simulink library "thermochemical"  (R2017b)
settings: Solver=VariableStepAuto  StartTime=0.0  StopTime=10.0  RelTol=1e-3
values from neighbouring files (symbols this model uses):
  c = conversion_factors()    [blk_clausius_clapeyron.m]    (also in blk_clausius_clapeyron_no_popup.m; blk_cold_room_closed_dry_air.m; blk_reactor_BaCl2_NH3_no_walls.m; blk_reactor_BaCl2_NH3_no_walls_state_space.m)
  cp = metal.cp    [blk_wall_simple.m]    (also in get_metal_properties.m = 390)
  fluid = get_param(blk,'fluid')    [blk_thermodynamic_properties_nonsaturated.m]    (also in blk_thermodynamic_properties_nonsaturated_interpreted.m; blk_thermodynamic_properties_saturated.m; blk_thermodynamic_properties_saturated_interpreted.m; blk_thermodynamic_properties_saturated_mix.m)
  gas = get_material_properties(x.gasName)    [blk_reactor_BaCl2_NH3_cylindrical_no_walls_fun1.m]
  h = get_param(gcb,'ObjectParameters')    [get_param_eval.m]
  rho = metal.rho    [blk_wall_simple.m]    (also in get_metal_properties.m = 8940)
  s = solve(eq,dx,'ReturnConditions',true)    [LMTD_inv.m]    (also in blk_wall_simple.m = get_param_eval(blk,'s'))
  u_gas_at_T_ref = -R * T_ref    [blk_reactor_BaCl2_NH3_no_walls.m]    (also in blk_reactor_BaCl2_NH3_no_walls_state_space.m)
undefined symbols (not defined in the file or in its folder): b_motor, BaCl2, beta, CoolProp, cP_binder, cP_gas, cP_s0, cv, dh_r_0, ENG, heat_exchanger_epsilonNTU_inv_simulink, heat_exchanger_epsilonNTU_simulink, J_motor, K_cin, kappa, Km_motor, La_motor, lookup2D_BreakPoint2, M_binder, N_binder, N_gas_free_volume_init, N_salt, NH3, nh3_v3, nu, P, phase, PID_D_motor, PID_I_motor, PID_P_motor, Ra_motor, Reactor_phase, T, T1, T2, T_init, Tr_init, Tr_ref, U_binder_at_Tr_ref, U_salt_at_X0_Tr_ref, Ur_init, V_void, Valve_regime, Vmax_motor, w_init_motor, X_init
libraries: thermochemical x247, simulink x54, dspsigops x3
(part 8 of 12)

== system thermochemical/Thermodynamic fluid properties/Thermodynamic property (non-saturated) (it uses CoolProp library)/Subsystem1 ==
  In1 : Inport
  In2 : Inport  Port=2
  Constant2 : Constant  Value=str2num(reciprocVar)
  CoolProp_function_call : MATLABFcn  MATLABFcn=CoolProp.PropsSI('Dmolar','T',u(1),'P',u(2)*100000,'Ammonia');
  Math Function : Math  Operator=reciprocal  SaturateOnIntegerOverflow=on
  Mux1 : Mux  Inputs=2
  switch2 : Switch  Criteria=u2 > Threshold
  Out1 : Outport
  wires:
  In2/1 -> Mux1/2
  In1/1 -> Mux1/1
  switch2/1 -> Out1/1
  Math Function/1 -> switch2/1
  Constant2/1 -> switch2/2
  CoolProp_function_call/1 -> Math Function/1, switch2/3
  Mux1/1 -> CoolProp_function_call/1

== system thermochemical/Thermodynamic fluid properties/Thermodynamic property (saturated)/Subsystem1 ==
  In1 : Inport
  look-up table 1D : Lookup_n-D  NumberOfTableDimensions=1  BreakpointsForDimension1=lookup1D_BreakPoint1  BreakpointsForDimension2=lookup2D_BreakPoint2  BreakpointsForDimension3=[5, 7]  BeginIndexSearchUsingPreviousIndexResult=on  Table=lookup1D_Data  ExtrapMethod=Clip  InternalRulePriority=Speed  RndMeth=Simplest  InputSameDT=on
  Out1 : Outport
  wires:
  In1/1 -> look-up table 1D/1
  look-up table 1D/1 -> Out1/1

== system thermochemical/Thermodynamic fluid properties/Thermodynamic property (saturated) (it uses CoolProp library)/Subsystem1 ==
  In1 : Inport
  Constant2 : Constant  Value=str2num(reciprocVar)
  CoolProp_function_call : MATLABFcn  MATLABFcn=CoolProp.PropsSI('P','T',u(1),'Q',0.5,'Ammonia')*1e-05;
  Math Function : Math  Operator=reciprocal  SaturateOnIntegerOverflow=on
  switch2 : Switch  Criteria=u2 > Threshold
  Out1 : Outport
  wires:
  In1/1 -> CoolProp_function_call/1
  switch2/1 -> Out1/1
  Math Function/1 -> switch2/1
  Constant2/1 -> switch2/2
  CoolProp_function_call/1 -> Math Function/1, switch2/3

== system thermochemical/Thermodynamic fluid properties/Thermodynamic property (saturated vapor-liquid mix)/Subsystem1 ==
  T(K) : Inport
  vapor quality (0..1) : Inport  Port=2
  1 : Constant
  Product : Product
  Product1 : Product
  Sum1 : Sum  Inputs=-+|
  Sum2 : Sum
  look-up table 1D : Lookup_n-D  NumberOfTableDimensions=1  BreakpointsForDimension1=fluid.sat.T  BreakpointsForDimension2=lookup2D_BreakPoint2  BreakpointsForDimension3=[5, 7]  BeginIndexSearchUsingPreviousIndexResult=on  Table=lookup1D_Data1  ExtrapMethod=Clip  InternalRulePriority=Speed  RndMeth=Simplest  InputSameDT=on
  look-up table 1D1 : Lookup_n-D  NumberOfTableDimensions=1  BreakpointsForDimension1=fluid.sat.T  BreakpointsForDimension2=lookup2D_BreakPoint2  BreakpointsForDimension3=[5, 7]  BeginIndexSearchUsingPreviousIndexResult=on  Table=lookup1D_Data2  ExtrapMethod=Clip  InternalRulePriority=Speed  RndMeth=Simplest  InputSameDT=on
  Out1 : Outport
  wires:
  Product1/1 -> Sum2/2
  1/1 -> Sum1/2
  Sum2/1 -> Out1/1
  Sum1/1 -> Product1/2  "1-Q"
  T(K)/1 -> look-up table 1D/1, look-up table 1D1/1
  look-up table 1D/1 -> Product1/1  "liquid"
  vapor quality (0..1)/1 -> Sum1/1, Product/2
  look-up table 1D1/1 -> Product/1  "vapor"
  Product/1 -> Sum2/1

== system thermochemical/Valves/Valve, gas, IEC 60534-2-1:2012 (exact)/Flow computation for compressible fluids, IEC 60534-2-1:2012 ==
  note: Valve flow model for compressible fluid,
      | according to IEC 60534-2-1:2012
  note: NOTE 2: for the 'regime' output to work properly, the model defines an enumerated type. This is done
      | inside the LoadFnc Callback of the model. (right click on the model -> Properties -> 'Callbacks' tab).
      | The enumerated type defined is the following:
      | Simulink.defineIntEnumType('Valve_regime',{'Open_NonChocked','Closed','Open_Chocked'},[1 0 -1])
  note: NOTE 1: Enumerations and Scopes
      | When a Scope block displays an enumerated signal, the vertical axis displays the names of
      | the enumerated values only if the scope was open during simulation. If you open the Scope
      | block for the first time before any simulation has occurred, or between simulations, the block
      | displays only numeric values.
  In1 : Inport
  In2 : Inport  Port=2
  In3 : Inport  Port=3
  In4 : Inport  Port=4
  In5 : Inport  Port=5
  Constant : Constant  Value=27.3
  Dead Zone : DeadZone  LowerValue=-Inf  UpperValue=1e-7  SaturateOnIntegerOverflow=on
  Display3 : Display
  Divide1 : Product  Inputs=***
  Divide2 : Product  Inputs=**
  Divide5 : Product  Inputs=***
  Sqrt : Sqrt  SaturateOnIntegerOverflow=on
  Subsystem : Subsystem
  Subsystem1 : Subsystem
  Valve regime : Subsystem
  Out1 : Outport
  Out2 : Outport  Port=2
  wires:
  Subsystem/1(non-chocked) -> Valve regime/2(In2)
  Divide2/1 -> Out1/1  "W (kg/h)"
  Sqrt/1 -> Divide2/2
  Divide1/1 -> Sqrt/1
  In5/1 -> Divide1/3  "rho upstream (kg/m3)"
  Divide5/1 -> Divide2/1  "N6 * Cv * Y"
  Constant/1 -> Divide5/3
  Subsystem1/1(Y) -> Divide5/2
  In1/1 -> Divide5/1, Dead Zone/1  "Cv"
  Subsystem/3(non-chocked1) -> Subsystem1/2(In2)
  Subsystem/2(non-chocked2) -> Divide1/1, Subsystem1/1(In1)  "x sizing"
  In2/1 -> Subsystem/3(P upstream (bar)1)  "gamma upstream (1)"
  In3/1 -> Subsystem/2(P upstream (bar)), Divide1/2  "P upstream (bar)"
  In4/1 -> Subsystem/1(P downstream (bar))  "P downstream (bar)"
  Valve regime/1(Out1) -> Out2/1, Display3/1  "regime"
  Dead Zone/1 -> Valve regime/1(In1)

== system thermochemical/Valves/Valve, gas, IEC 60534-2-1:2012 (modified ideal gas approx.)/Glow computation for compressible fluids, IEC 60534-2-1:2012 (modified ideal gas assumption) ==
  note: NOTE 1: Enumerations and Scopes
      | When a Scope block displays an enumerated signal, the vertical axis displays the names of
      | the enumerated values only if the scope was open during simulation. If you open the Scope
      | block for the first time before any simulation has occurred, or between simulations, the block
      | displays only numeric values.
  note: NOTE 2: for the 'regime' output to work properly, the model defines an enumerated type. This is done
      | inside the LoadFnc Callback of the model. (right click on the model -> Properties -> 'Callbacks' tab).
      | The enumerated type defined is the following:
      | Simulink.defineIntEnumType('Valve_regime',{'Open_NonChocked','Closed','Open_Chocked'},[1 0 -1])
  note: Valve flow model for compressible fluid,
      | according to IEC 60534-2-1:2012
      | (with modified ideal gas approximation)
  In1 : Inport
  In3 : Inport  Port=2
  In4 : Inport  Port=3
  In6 : Inport  Port=4
  In2 : Inport  Port=5
  In5 : Inport  Port=6
  gamma upstream (1) : Inport  Port=7
  Constant : Constant  Value=417
  Dead Zone : DeadZone  LowerValue=-Inf  UpperValue=1e-7  SaturateOnIntegerOverflow=on
  Display3 : Display
  Divide1 : Product  Inputs=*///
  Divide2 : Product  Inputs=**
  Divide5 : Product  Inputs=****
  Sqrt : Sqrt  SaturateOnIntegerOverflow=on
  Subsystem : Subsystem
  Subsystem1 : Subsystem
  Valve regime : Subsystem
  Out1 : Outport
  Out2 : Outport  Port=2
  wires:
  Dead Zone/1 -> Valve regime/1(In1)
  Valve regime/1(Out1) -> Display3/1, Out2/1  "regime"
  In4/1 -> Subsystem/1(P downstream (bar))  "P downstream (bar)"
  In3/1 -> Divide5/4, Subsystem/2(P upstream (bar))  "P upstream (bar)"
  In2/1 -> Subsystem/3(P upstream (bar)1)  "gamma upstream (1)"
  Subsystem/2(non-chocked2) -> Subsystem1/1(In1), Divide1/1  "x sizing"
  Subsystem/3(non-chocked1) -> Subsystem1/2(In2)
  In1/1 -> Dead Zone/1, Divide5/1  "Cv"
  Subsystem1/1(Y) -> Divide5/2
  Constant/1 -> Divide5/3
  Divide5/1 -> Divide2/1  "N7 * Cv * Y * P1"
  In5/1 -> Divide1/4  "compressibility factor Z (1)"
  Divide1/1 -> Sqrt/1
  Sqrt/1 -> Divide2/2
  Divide2/1 -> Out1/1  "Qs (std m3/h) @ [60°F,1atm]"
  Subsystem/1(non-chocked) -> Valve regime/2(In2)
  gamma upstream (1)/1 -> Divide1/2  "molecular weight ratio Gg (Mgas/Mair) (1)"
  In6/1 -> Divide1/3  "T upstream (K)"

== system thermochemical/Valves/Valve, gas, Swagelok model/Gas flow computation ('Swagelok' equations) ==
  note: NOTE 2: for the 'regime' output to work properly, the model defines an enumerated type. This is done
      | inside the LoadFnc Callback of the model. (right click on the model -> Properties -> 'Callbacks' tab).
      | The enumerated type defined is the following:
      | Simulink.defineIntEnumType('Valve_regime',{'Open_Subcritical','Closed','Open_Supercritical'},[1 0 -1])
  note: NOTE 1: Enumerations and Scopes
      | When a Scope block displays an enumerated signal, the vertical axis displays the names of
      | the enumerated values only if the scope was open during simulation. If you open the Scope
      | block for the first time before any simulation has occurred, or between simulations, the block
      | displays only numeric values.
  In1 : Inport
  In2 : Inport  Port=2
  In3 : Inport  Port=3
  In4 : Inport  Port=4
  "Air density (kg/m3) at 'old' standard conditions (60°F, 1atm)" : Constant  Value=1.2232
  Dead Zone : DeadZone  LowerValue=-Inf  UpperValue=1e-7  SaturateOnIntegerOverflow=on
  Display3 : Display
  Divide2 : Product  Inputs=*/
  Gain1 : Gain  Gain=1/2
  "Gas density (kg/m3) at 'old' standard conditions (60°F, 1atm)" : Constant  Value=rho_gas_60F_1atm_kg_m3
  Pressure conversion : thermochemical/Conversions/Pressure conversion  sel=bar --> psi
      settings: SourceProductName=@ Thermochemical
  Pressure conversion1 : thermochemical/Conversions/Pressure conversion  sel=bar --> psi
      settings: SourceProductName=@ Thermochemical
  Sub-critical (P2 > 1/2 P1) : Subsystem
  Sum1 : Sum  Inputs=-+|
  Sum2 : Sum  Inputs=+-
  Super-critical (P2 < 1/2 P1) : Subsystem
  Switch : Switch  Criteria=u2 > Threshold
  Temperature conversion : thermochemical/Conversions/Temperature conversion  sel=K --> °R
      settings: SourceProductName=@ Thermochemical
  Valve regime : Subsystem
  Out1 : Outport
  Out2 : Outport  Port=2
  wires:
  Super-critical (P2 < 1/2 P1)/1(c) -> Switch/3  "super-critical"
  Sum1/1 -> Switch/2, Valve regime/1(In2)  "P2 - 1/2 P1"
  Gain1/1 -> Sum1/1
  Sub-critical (P2 > 1/2 P1)/1(c) -> Switch/1  "sub-critical"
  In4/1 -> Sum1/2, Pressure conversion1/1  "P downstream (bar)"
  In3/1 -> Gain1/1, Pressure conversion/1  "P upstream (bar)"
  In2/1 -> Temperature conversion/1  "T upstream (K)"
  Pressure conversion/1 -> Sum2/1, Super-critical (P2 < 1/2 P1)/4(P1), Sub-critical (P2 > 1/2 P1)/4(P1)
  Pressure conversion1/1 -> Sum2/2
  "Gas density (kg/m3) at 'old' standard conditions (60°F, 1atm)"/1 -> Divide2/1
  "Air density (kg/m3) at 'old' standard conditions (60°F, 1atm)"/1 -> Divide2/2
  Divide2/1 -> Super-critical (P2 < 1/2 P1)/1(Ggas), Sub-critical (P2 > 1/2 P1)/1(Ggas)  "Ggas"
  Temperature conversion/1 -> Super-critical (P2 < 1/2 P1)/3(T1 (°R)), Sub-critical (P2 > 1/2 P1)/3(T1 (°R))  "T1 (°R)"
  Sum2/1 -> Sub-critical (P2 > 1/2 P1)/5(dP)
  In1/1 -> Dead Zone/1, Super-critical (P2 < 1/2 P1)/2(Ggas1), Sub-critical (P2 > 1/2 P1)/2(Ggas1)  "Cv"
  Switch/1 -> Out1/1, Display3/1  "SCFH"
  Valve regime/1(Out1) -> Out2/1  "regime"
  Dead Zone/1 -> Valve regime/2(In1)

== system thermochemical/Valves/Valve, liquid (chocked condition not implemented)/Volume flow computation ==
  note: NOTE 2: for the 'regime' output to work properly, the model defines an enumerated type. This is done
      | inside the LoadFnc Callback of the model. (right click on the model -> Properties -> 'Callbacks' tab).
      | The enumerated type defined is the following:
      | Simulink.defineIntEnumType('Valve_regime',{'Open','Closed'},[1 0])
  note: NOTE 1: Enumerations and Scopes
      | When a Scope block displays an enumerated signal, the vertical axis displays the names of
      | the enumerated values only if the scope was open during simulation. If you open the Scope
      | block for the first time before any simulation has occurred, or between simulations, the block
      | displays only numeric values.
  In1 : Inport
  In3 : Inport  Port=2
  In4 : Inport  Port=3
  In2 : Inport  Port=4
  Dead Zone : DeadZone  LowerValue=-Inf  UpperValue=1e-7  SaturateOnIntegerOverflow=on
  Display1 : Display
  Display3 : Display
  Divide2 : Product  Inputs=/*
  Pressure conversion : thermochemical/Conversions/Pressure conversion  sel=bar --> psi
      settings: SourceProductName=@ Thermochemical
  Sum2 : Sum  Inputs=+-
  Turbulent & non-choked flow conditions : Subsystem
  Valve regime : Subsystem
  "Water density (kg/m3) at 'old' standard conditions (60°F, 1atm)" : Constant  Value=1e3
  Out1 : Outport
  Out2 : Outport  Port=2
  wires:
  In4/1 -> Sum2/2  "P downstream (bar)"
  In3/1 -> Sum2/1  "P upstream (bar)"
  "Water density (kg/m3) at 'old' standard conditions (60°F, 1atm)"/1 -> Divide2/1
  Divide2/1 -> Turbulent & non-choked flow conditions/1(Ggas)  "G (dimensionless)"
  Sum2/1 -> Display1/1, Pressure conversion/1
  In1/1 -> Dead Zone/1, Turbulent & non-choked flow conditions/3(Ggas1)  "Cv"
  Turbulent & non-choked flow conditions/1(c) -> Out1/1, Display3/1  "US gpm"
  Valve regime/1(Out1) -> Out2/1  "regime"
  Dead Zone/1 -> Valve regime/1(In1)
  In2/1 -> Divide2/2  "rho uptream (kg/m3) at process T,P conditions"
  Pressure conversion/1 -> Turbulent & non-choked flow conditions/2(dP)

== system thermochemical/Valves/Valve, liquid, IEC 60534-2-1:2012/Flow computation for incompressible fluids, IEC 60534-2-1:2012 ==
  note: NOTE 1: Enumerations and Scopes
      | When a Scope block displays an enumerated signal, the vertical axis displays the names of
      | the enumerated values only if the scope was open during simulation. If you open the Scope
      | block for the first time before any simulation has occurred, or between simulations, the block
      | displays only numeric values.
  note: NOTE 2: for the 'regime' output to work properly, the model defines an enumerated type. This is done
      | inside the LoadFnc Callback of the model. (right click on the model -> Properties -> 'Callbacks' tab).
      | The enumerated type defined is the following:
      | Simulink.defineIntEnumType('Valve_regime',{'Open_NonChocked','Closed','Open_Chocked'},[1 0 -1])
  note: Valve flow model for incompressible fluid,
      | according to IEC 60534-2-1:2012
  In1 : Inport
  In3 : Inport  Port=2
  In4 : Inport  Port=3
  P upstream (bar)2 : Inport  Port=4
  P upstream (bar)1 : Inport  Port=5
  In5 : Inport  Port=6
  Constant : Constant  Value=1000
  Dead Zone : DeadZone  LowerValue=-Inf  UpperValue=1e-7  SaturateOnIntegerOverflow=on
  Display3 : Display
  Divide1 : Product  Inputs=*/
  Divide2 : Product  Inputs=**
  Divide3 : Product  Inputs=*/
  Pressure conversion : thermochemical/Conversions/Pressure conversion  sel=bar --> psi
      settings: SourceProductName=@ Thermochemical
  Sqrt : Sqrt  SaturateOnIntegerOverflow=on
  Valve regime : Subsystem
  dP sizing computation : Subsystem
  Out1 : Outport
  Out2 : Outport  Port=2
  wires:
  Dead Zone/1 -> Valve regime/1(In1)
  Valve regime/1(Out1) -> Display3/1, Out2/1  "regime"
  In4/1 -> dP sizing computation/2(P upstream (bar)3)  "P downstream (bar)"
  In3/1 -> dP sizing computation/1(P upstream (bar))  "P upstream (bar)"
  dP sizing computation/2(non-chocked2) -> Pressure conversion/1  "dP sizing (bar)"
  In1/1 -> Divide2/1, Dead Zone/1  "Cv"
  Divide1/1 -> Sqrt/1
  Sqrt/1 -> Divide2/2
  Divide2/1 -> Out1/1  "Q (US gpm)"
  dP sizing computation/1(non-chocked) -> Valve regime/2(In2)
  P upstream (bar)1/1 -> dP sizing computation/4(P upstream (bar)1)  "Pc: absolute thermodynamic  critical pressure (bar)"
  P upstream (bar)2/1 -> dP sizing computation/3(P upstream (bar)2)  "Pv: absolute vapor pressure  of liquid at T upstream (bar)"
  Constant/1 -> Divide3/2  "rho water @ [60°F,1atm] (kg/m3)"
  In5/1 -> Divide3/1  "rho upstream (kg/m3)"
  Divide3/1 -> Divide1/2  "rho1/rho0"
  Pressure conversion/1 -> Divide1/1  "dP sizing (psi)"

== system thermochemical/Walls/Fin efficiency/Square root ==
  In1 : Inport
  Constant : Constant  Value=0.5
  Math Function : Math  Operator=pow  SaturateOnIntegerOverflow=on
  m : Outport
  wires:
  In1/1 -> Math Function/1  "u"
  Constant/1 -> Math Function/2
  Math Function/1 -> m/1  "y"

== system thermochemical/Walls/Wall, tube with//without fins/Subsystem ==
  In1 : Inport
  In2 : Inport  Port=2
  In3 : Inport  Port=3
  Gain2 : Gain  Gain=1e-3
  Gain3 : Gain  Gain=pi
  Gain4 : Gain  Gain=2
  Product2 : Product
  Sum : Sum  Inputs=+-
  Inner area (m2) : Outport
  wires:
  Sum/1 -> Gain2/1
  In3/1 -> Product2/2  "L_m"
  Product2/1 -> Inner area (m2)/1  "Inner area (m²)"
  In2/1 -> Gain4/1  "e_mm"
  In1/1 -> Sum/1  "OD_mm"
  Gain2/1 -> Gain3/1  "Inner diameter (m)"
  Gain3/1 -> Product2/1
  Gain4/1 -> Sum/2

== system thermochemical/Walls/Wall, tube with//without fins/Subsystem1 ==
  Product3 : Product  Inputs=3
  Product4 : Product  Inputs=3
  Subsystem2 : Subsystem
  Sum1 : Sum
  s1 : Constant  Value=cp_fin
  s15 : Constant  Value=rho_fin
  s16 : Constant  Value=cp_tube
  s17 : Constant  Value=rho_tube
  (m*Cp) fins + (m*Cp) tube : Outport
  wires:
  Subsystem2/1(Total tube effective finned area (m2)) -> Product3/3
  Product4/1 -> Sum1/2  "m * Cp tube"
  Sum1/1 -> (m*Cp) fins + (m*Cp) tube/1  "(m*Cp) fins + (m*Cp) tube"
  s15/1 -> Product3/1
  Product3/1 -> Sum1/1  "m * Cp fins"
  Subsystem2/2(Inner area (m2)) -> Product4/1
  s17/1 -> Product4/3
  s16/1 -> Product4/2
  s1/1 -> Product3/2

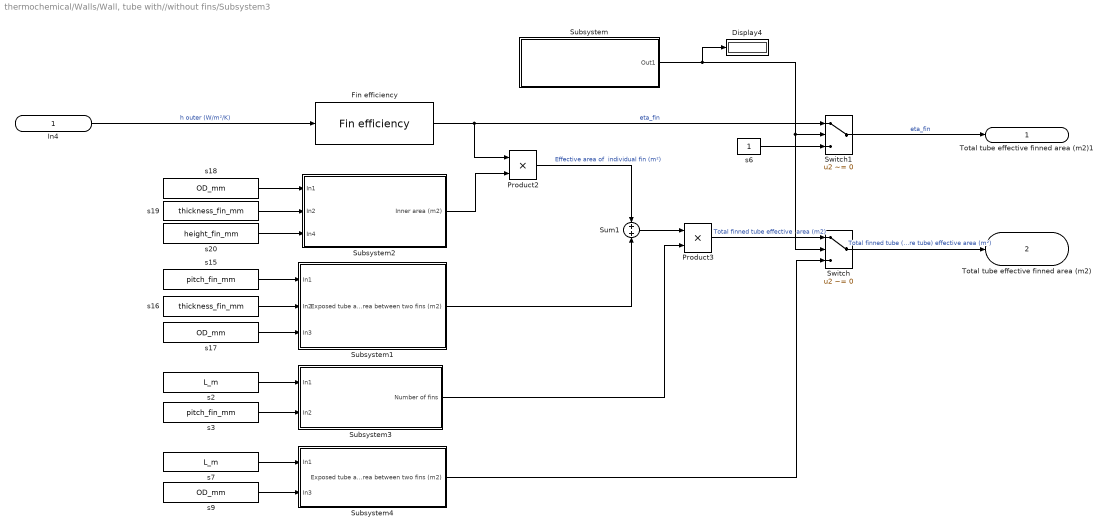
== system thermochemical/Walls/Wall, tube with//without fins/Subsystem3 ==
  In4 : Inport
  Display4 : Display
  Fin efficiency : thermochemical/Walls/Fin efficiency  D_mm=OD_mm  height_fin_mm=max(height_fin_mm, 1e-7)  thickness_fin_mm=max(thickness_fin_mm, 1e-7)  lambda=max(lambda_fin, 1e-7)
      settings: SourceProductName=@ Thermochemical
  Product2 : Product
  Product3 : Product
  Subsystem : Subsystem
  Subsystem1 : Subsystem
  Subsystem2 : Subsystem
  Subsystem3 : Subsystem
  Subsystem4 : Subsystem
  Sum1 : Sum
  Switch : Switch  Criteria=u2 ~= 0
  Switch1 : Switch  Criteria=u2 ~= 0
  s15 : Constant  Value=pitch_fin_mm
  s16 : Constant  Value=thickness_fin_mm
  s17 : Constant  Value=OD_mm
  s18 : Constant  Value=OD_mm
  s19 : Constant  Value=thickness_fin_mm
  s2 : Constant  Value=L_m
  s20 : Constant  Value=height_fin_mm
  s3 : Constant  Value=pitch_fin_mm
  s6 : Constant
  s7 : Constant  Value=L_m
  s9 : Constant  Value=OD_mm
  Total tube effective finned area (m2)1 : Outport
  Total tube effective finned area (m2) : Outport  Port=2
  wires:
  Subsystem4/1(Exposed tube area between two fins (m2)) -> Switch/3
  s7/1 -> Subsystem4/1(In1)
  s9/1 -> Subsystem4/2(In3)
  Product3/1 -> Switch/1  "Total finned tube effective  area (m2)"
  s6/1 -> Switch1/3
  Switch1/1 -> Total tube effective finned area (m2)1/1  "eta_fin"
  Sum1/1 -> Product3/1
  s17/1 -> Subsystem1/3(In3)
  s16/1 -> Subsystem1/2(In2)
  s15/1 -> Subsystem1/1(In1)
  s2/1 -> Subsystem3/1(In1)
  s3/1 -> Subsystem3/2(In2)
  In4/1 -> Fin efficiency/1  "h outer (W/m²/K)"
  Switch/1 -> Total tube effective finned area (m2)/1  "Total finned tube (or bare tube) effective area (m²)"
  s19/1 -> Subsystem2/2(In2)
  s18/1 -> Subsystem2/1(In1)
  s20/1 -> Subsystem2/3(In4)
  Subsystem1/1(Exposed tube area between two fins (m2)) -> Sum1/2
  Subsystem3/1(Number of fins) -> Product3/2
  Product2/1 -> Sum1/1  "Effective area of  individual fin (m²)"
  Fin efficiency/1 -> Switch1/1, Product2/1  "eta_fin"
  Subsystem2/1(Inner area (m2)) -> Product2/2
  Subsystem/1(Out1) -> Switch/2, Switch1/2, Display4/1

== system thermochemical/Walls/Wall, tube with//without fins, with internal heat production/Subsystem ==
  In1 : Inport
  In2 : Inport  Port=2
  In3 : Inport  Port=3
  Gain1 : Gain  Gain=2
  Gain2 : Gain  Gain=1e-3
  Gain3 : Gain  Gain=pi
  Product2 : Product
  Sum : Sum  Inputs=+-
  Inner area (m2) : Outport
  wires:
  Gain3/1 -> Product2/1
  Gain2/1 -> Gain3/1  "Inner diameter (m)"
  In1/1 -> Sum/1  "OD_mm"
  In2/1 -> Gain1/1  "e_mm"
  Product2/1 -> Inner area (m2)/1  "Inner area (m²)"
  In3/1 -> Product2/2  "L_m"
  Sum/1 -> Gain2/1
  Gain1/1 -> Sum/2

== system thermochemical/Walls/Wall, tube with//without fins, with internal heat production/Subsystem1 ==
  Product3 : Product  Inputs=3
  Product4 : Product  Inputs=3
  Subsystem2 : Subsystem
  Sum1 : Sum
  s1 : Constant  Value=cp_fin
  s15 : Constant  Value=rho_fin
  s16 : Constant  Value=cp_tube
  s17 : Constant  Value=rho_tube
  (m*Cp) fins + (m*Cp) tube : Outport
  wires:
  s1/1 -> Product3/2
  s16/1 -> Product4/2
  s17/1 -> Product4/3
  Subsystem2/2(Inner area (m2)) -> Product4/1
  Product3/1 -> Sum1/1  "m * Cp fins"
  s15/1 -> Product3/1
  Sum1/1 -> (m*Cp) fins + (m*Cp) tube/1  "(m*Cp) fins + (m*Cp) tube"
  Product4/1 -> Sum1/2  "m * Cp tube"
  Subsystem2/1(Total tube effective finned area (m2)) -> Product3/3

== system thermochemical/Walls/Wall, tube with//without fins, with internal heat production/Subsystem3 ==
  In4 : Inport
  Display4 : Display
  Fin efficiency : thermochemical/Walls/Fin efficiency  D_mm=OD_mm  height_fin_mm=max(height_fin_mm, 1e-7)  thickness_fin_mm=max(thickness_fin_mm, 1e-7)  lambda=max(lambda_fin, 1e-7)
      settings: SourceProductName=@ Thermochemical
  Product2 : Product
  Product3 : Product
  Subsystem : Subsystem
  Subsystem1 : Subsystem
  Subsystem2 : Subsystem
  Subsystem3 : Subsystem
  Subsystem4 : Subsystem
  Sum1 : Sum
  Switch : Switch  Criteria=u2 ~= 0
  Switch1 : Switch  Criteria=u2 ~= 0
  s15 : Constant  Value=pitch_fin_mm
  s16 : Constant  Value=thickness_fin_mm
  s17 : Constant  Value=OD_mm
  s18 : Constant  Value=OD_mm
  s19 : Constant  Value=thickness_fin_mm
  s2 : Constant  Value=L_m
  s20 : Constant  Value=height_fin_mm
  s3 : Constant  Value=pitch_fin_mm
  s6 : Constant
  s7 : Constant  Value=L_m
  s9 : Constant  Value=OD_mm
  Total tube effective finned area (m2)1 : Outport
  Total tube effective finned area (m2) : Outport  Port=2
  wires:
  Subsystem/1(Out1) -> Display4/1, Switch1/2, Switch/2
  Subsystem2/1(Inner area (m2)) -> Product2/2
  Fin efficiency/1 -> Product2/1, Switch1/1  "eta_fin"
  Product2/1 -> Sum1/1  "Effective area of  individual fin (m²)"
  Subsystem3/1(Number of fins) -> Product3/2
  Subsystem1/1(Exposed tube area between two fins (m2)) -> Sum1/2
  s20/1 -> Subsystem2/3(In4)
  s18/1 -> Subsystem2/1(In1)
  s19/1 -> Subsystem2/2(In2)
  Switch/1 -> Total tube effective finned area (m2)/1  "Total finned tube (or bare tube) effective area (m²)"
  In4/1 -> Fin efficiency/1  "h outer (W/m²/K)"
  s3/1 -> Subsystem3/2(In2)
  s2/1 -> Subsystem3/1(In1)
  s15/1 -> Subsystem1/1(In1)
  s16/1 -> Subsystem1/2(In2)
  s17/1 -> Subsystem1/3(In3)
  Sum1/1 -> Product3/1
  Switch1/1 -> Total tube effective finned area (m2)1/1  "eta_fin"
  s6/1 -> Switch1/3
  Product3/1 -> Switch/1  "Total finned tube effective  area (m2)"
  s9/1 -> Subsystem4/2(In3)
  s7/1 -> Subsystem4/1(In1)
  Subsystem4/1(Exposed tube area between two fins (m2)) -> Switch/3

== system thermochemical/Control volumes/Two-phase saturated fluid control volume (without walls)/Internal energy differential equation/HX energy rate balance ==
  In1 : Inport
  In2 : Inport  Port=2
  In3 : Inport  Port=3
  In5 : Inport  Port=4
  In4 : Inport  Port=5
  In7 : Inport  Port=6
  In6 : Inport  Port=7
  Check Dynamic Lower Bound : simulink/Model Verification/Check Dynamic  Lower Bound  Description=min < u  Enabled=on  stopWhenAssertionFail=on  export=off  icon=graphic
      settings: SourceProductName=Simulink  SourceProductBaseCode=SL
  Check Dynamic Lower Bound1 : simulink/Model Verification/Check Dynamic  Lower Bound  Description=min < u  Enabled=on  stopWhenAssertionFail=on  export=off  icon=graphic
      settings: SourceProductName=Simulink  SourceProductBaseCode=SL
  Check Dynamic Lower Bound2 : simulink/Model Verification/Check Dynamic  Lower Bound  Description=min < u  Enabled=on  stopWhenAssertionFail=on  export=off  icon=graphic
      settings: SourceProductName=Simulink  SourceProductBaseCode=SL
  Product1 : Product
  Product2 : Product
  Product3 : Product
  Sum13 : Sum  Inputs=++--
  dn_gas1 : Constant  Value=-1e-5
  dn_gas2 : Constant  Value=-1e-5
  dn_gas3 : Constant  Value=-1e-5
  Out1 : Outport
  wires:
  Sum13/1 -> Out1/1  "dU/dt hx (J/sec)"
  Product2/1 -> Sum13/2
  Product1/1 -> Sum13/3
  Product3/1 -> Sum13/4
  In4/1 -> Check Dynamic Lower Bound1/2, Product1/2  "dn/dt vap,out (mol/sec)"
  In3/1 -> Check Dynamic Lower Bound/2, Product2/2  "dn/dt in (mol/sec)"
  In7/1 -> Product3/1  "h liq (J/mol)"
  In2/1 -> Product2/1  "h in (J/mol)"
  In1/1 -> Sum13/1  "q wall → hx (W)"
  In5/1 -> Product1/1  "h vap (J/mol)"
  In6/1 -> Check Dynamic Lower Bound2/2, Product3/2  "dn/dt liq,out (mol/sec)"
  dn_gas2/1 -> Check Dynamic Lower Bound1/1
  dn_gas3/1 -> Check Dynamic Lower Bound2/1
  dn_gas1/1 -> Check Dynamic Lower Bound/1

== system thermochemical/Control volumes/Two-phase saturated fluid control volume (without walls) (without algebraic loop)/Two-phase control volume state-space functions/f1 ==
  In6 : Inport
  In1 : Inport  Port=2
  Demux : Demux  Outputs=2
  Demux1 : Demux  Outputs=5
  HX energy rate balance : thermochemical/Control volumes/Two-phase saturated fluid control volume (without walls)/Internal energy differential equation/HX energy rate balance
      settings: SourceProductName=@ Thermochemical
  Product : Product  Inputs=/*
  Product1 : Product  Inputs=**
  Subsystem : Subsystem
  Subsystem1 : Subsystem
  Sum : Sum  Inputs=-+
  Thermodynamic property (saturated) : thermochemical/Thermodynamic fluid properties/Thermodynamic  property (saturated)  sel=h(T) vap. (J/mol)  fluid=fluid  lookup1D_BreakPoint1=fluid.sat.T  lookup1D_Data=fluid.sat.vap.h_molar
      settings: SourceProductName=@ Thermochemical
  Thermodynamic property (saturated)1 : thermochemical/Thermodynamic fluid properties/Thermodynamic  property (saturated)  sel=h(T) liq. (J/mol)  fluid=fluid  lookup1D_BreakPoint1=fluid.sat.T  lookup1D_Data=fluid.sat.liq.h_molar
      settings: SourceProductName=@ Thermochemical
  f2 : thermochemical/Control volumes/Two-phase saturated fluid control volume (without walls) (without algebraic loop)/Two-phase control volume state-space functions/f2
      settings: SourceProductName=@ Thermochemical
  Out2 : Outport
  wires:
  Product/1 -> Out2/1  "dT/dt (K/sec)"
  Demux/2 -> Subsystem/2(In3), Subsystem1/2(In3)  "x(2) = v (mol)"
  In6/1 -> f2/1, Demux/1  "X"
  In1/1 -> f2/2, Demux1/1  "U"
  Demux/1 -> Thermodynamic property (saturated)1/1, Thermodynamic property (saturated)/1, Subsystem/1(In2), Subsystem1/1(In2)  "x(1) = T (K)"
  HX energy rate balance/1 -> Sum/2  "dU/dt hx (J/sec)"
  Subsystem/1(Out1) -> Product1/1  "∂U/∂v|T (J.mol/m³)"
  Subsystem1/1(Out1) -> Product/1  "∂U/∂T|v (J/K)"
  f2/1 -> Product1/2  "dv/dt (m³/mol/sec)"
  Sum/1 -> Product/2
  Product1/1 -> Sum/1
  Demux1/1 -> HX energy rate balance/1  "q wall → exchanger (W)"
  Demux1/3 -> HX energy rate balance/3  "dn/dt in (mol/sec)"
  Demux1/4 -> HX energy rate balance/5  "dn/dt vap,out (mol/sec)"
  Demux1/2 -> HX energy rate balance/2  "h in (J/mol)"
  Demux1/5 -> HX energy rate balance/7  "dn/dt liq,out (mol/sec)"
  Thermodynamic property (saturated)/1 -> HX energy rate balance/4
  Thermodynamic property (saturated)1/1 -> HX energy rate balance/6

== system thermochemical/Control volumes/Two-phase saturated fluid control volume (without walls) (without algebraic loop)/Two-phase control volume state-space functions/f2 ==
  In6 : Inport
  In2 : Inport  Port=2
  2 : Constant  Value=V
  Demux : Demux  Outputs=2
  Demux2 : Demux  Outputs=5
  Gain : Gain  Gain=-1
  Math Function : Math  Operator=square  SaturateOnIntegerOverflow=on
  Product : Product  Inputs=*/
  Product1 : Product  Inputs=**
  Sum2 : Sum  Inputs=+--
  Terminator1 : Terminator
  Terminator5 : Terminator
  Terminator6 : Terminator
  Out2 : Outport
  wires:
  Demux/1 -> Terminator5/1  "x(1) = T (K)"
  In6/1 -> Demux/1  "X"
  Product1/1 -> Gain/1
  Demux/2 -> Math Function/1  "x(2) = v (mol)"
  Sum2/1 -> Product1/2
  Math Function/1 -> Product/1
  2/1 -> Product/2
  Product/1 -> Product1/1
  Demux2/2 -> Terminator6/1  "h in (J/mol)"
  Demux2/3 -> Sum2/1  "dn/dt in (mol/sec)"
  Demux2/1 -> Terminator1/1  "q wall → exchanger (W)"
  Demux2/5 -> Sum2/3  "dn/dt liq,out (mol/sec)"
  Demux2/4 -> Sum2/2  "dn/dt vap,out (mol/sec)"
  In2/1 -> Demux2/1  "U"
  Gain/1 -> Out2/1  "dv/dt (m³/mol/sec)"

== system thermochemical/Heat exchangers/Heat Exchanger, e-NTU method (UA input) Loop 2: water/Subsystem/NTU as a function of flow configuration ==
  In1 : Inport
  In6 : Inport  Port=2
  Flow type (numeric) : Constant  Value=0
  MATLAB Function : MATLAB Function  TreatAsAtomicUnit=on
  Q HX2 (W)8 : Outport
  wires:
  Flow type (numeric)/1 -> MATLAB Function/3(flowType_numeric)
  MATLAB Function/1(epsilon) -> Q HX2 (W)8/1  "epsilon (0..1)"
  In1/1 -> MATLAB Function/2(Cr)  "Cr (0..1)"
  In6/1 -> MATLAB Function/1(NTU)  "NTU (1)"

== system thermochemical/Heat exchangers/Heat Exchanger, e-NTU method (UA input) Loop 2: water/Subsystem/Subsystem1 ==
  In1 : Inport
  In2 : Inport  Port=2
  In3 : Inport  Port=3
  In4 : Inport  Port=4
  In5 : Inport  Port=5
  Average : Subsystem
  Display1 : Display
  Display6 : Display
  Divide : Product  Inputs=/*
  MinMax : MinMax  Function=max  Inputs=2
  MinMax1 : MinMax  Inputs=2
  Product : Product
  Product1 : Product
  Thermodynamic property (non-saturated) : thermochemical/Thermodynamic fluid properties/Thermodynamic  property (non-saturated)  sel=cp(T,P)  fluid=fluid  reciprocVar=-1  lookup2D_BreakPoint1=fluid.no_sat.T_P_indep.var_indep.T  lookup2D_BreakPoint2=fluid.no_sat.T_P_indep.var_indep.P  lookup2D_Data=fluid.no_sat.T_P_indep.var_dep.Cp_molar
      settings: SourceProductName=@ Thermochemical
  cp water (J/mol) : Constant  Value=cp_water_J_K_mol
  Q HX2 (W)1 : Outport
  Q HX2 (W)7 : Outport  Port=2
  Q HX2 (W)2 : Outport  Port=3
  Q HX2 (W)3 : Outport  Port=4
  wires:
  MinMax1/1 -> Divide/2, Q HX2 (W)1/1  "Cmin (W/K)"
  Product1/1 -> MinMax1/2, MinMax/2, Q HX2 (W)3/1  "C2 (W/K)"
  In5/1 -> Product1/2  "dn/dt 2 (mol/sec)"
  Divide/1 -> Q HX2 (W)7/1  "Cr"
  MinMax/1 -> Divide/1  "Cmax (W/K)"
  cp water (J/mol)/1 -> Product1/1  "cp2 avg (J/K·mol)"
  Product/1 -> MinMax/1, MinMax1/1, Q HX2 (W)2/1  "C1 (W/K)"
  In3/1 -> Thermodynamic property (non-saturated)/2  "P1 in = P1 out (bar)"
  Thermodynamic property (non-saturated)/1 -> Product/1, Display1/1  "cp1 avg (J/K/mol)"
  Average/1(Out1) -> Thermodynamic property (non-saturated)/1, Display6/1  "T1 avg"
  In4/1 -> Product/2  "dn/dt 1 (mol/sec)"
  In2/1 -> Average/2(In2)  "T1 out (K)"
  In1/1 -> Average/1(In1)  "T1 in (K)"

== system thermochemical/Heat exchangers/Heat Exchanger, e-NTU method (epsilon input) Loop 2: water/Subsystem/NTU as a function of flow configuration ==
  In1 : Inport
  In6 : Inport  Port=2
  Flow type (numeric) : Constant  Value=0
  MATLAB Function : MATLAB Function  TreatAsAtomicUnit=on
  Q HX2 (W)8 : Outport
  wires:
  In6/1 -> MATLAB Function/1(epsilon)  "epsilon (0..1)"
  In1/1 -> MATLAB Function/2(Cr)  "Cr (0..1)"
  MATLAB Function/1(NTU) -> Q HX2 (W)8/1  "NTU (1)"
  Flow type (numeric)/1 -> MATLAB Function/3(flowType_numeric)

== system thermochemical/Heat exchangers/Heat Exchanger, e-NTU method (epsilon input) Loop 2: water/Subsystem/Subsystem1 ==
  In1 : Inport
  In2 : Inport  Port=2
  In3 : Inport  Port=3
  In4 : Inport  Port=4
  In5 : Inport  Port=5
  Average : Subsystem
  Display1 : Display
  Display6 : Display
  Divide : Product  Inputs=/*
  MinMax : MinMax  Function=max  Inputs=2
  MinMax1 : MinMax  Inputs=2
  Product : Product
  Product1 : Product
  Thermodynamic property (non-saturated) : thermochemical/Thermodynamic fluid properties/Thermodynamic  property (non-saturated)  sel=cp(T,P)  fluid=fluid  reciprocVar=-1  lookup2D_BreakPoint1=fluid.no_sat.T_P_indep.var_indep.T  lookup2D_BreakPoint2=fluid.no_sat.T_P_indep.var_indep.P  lookup2D_Data=fluid.no_sat.T_P_indep.var_dep.Cp_molar
      settings: SourceProductName=@ Thermochemical
  cp water (J/mol) : Constant  Value=cp_water_J_K_mol
  Q HX2 (W)1 : Outport
  Q HX2 (W)7 : Outport  Port=2
  Q HX2 (W)2 : Outport  Port=3
  Q HX2 (W)3 : Outport  Port=4
  wires:
  In1/1 -> Average/1(In1)  "T1 in (K)"
  In2/1 -> Average/2(In2)  "T1 out (K)"
  In4/1 -> Product/2  "dn/dt 1 (mol/sec)"
  Average/1(Out1) -> Display6/1, Thermodynamic property (non-saturated)/1  "T1 avg"
  Thermodynamic property (non-saturated)/1 -> Display1/1, Product/1  "cp1 avg (J/K/mol)"
  In3/1 -> Thermodynamic property (non-saturated)/2  "P1 in = P1 out (bar)"
  Product/1 -> Q HX2 (W)2/1, MinMax1/1, MinMax/1  "C1 (W/K)"
  cp water (J/mol)/1 -> Product1/1  "cp2 avg (J/K·mol)"
  MinMax/1 -> Divide/1  "Cmax (W/K)"
  Divide/1 -> Q HX2 (W)7/1  "Cr"
  In5/1 -> Product1/2  "dn/dt 2 (mol/sec)"
  Product1/1 -> Q HX2 (W)3/1, MinMax/2, MinMax1/2  "C2 (W/K)"
  MinMax1/1 -> Q HX2 (W)1/1, Divide/2  "Cmin (W/K)"

== system thermochemical/Reactors/Reactor, BaCl2//NH3, state-space form, [Tr, Ng, X] as state variables, no algebraic loops, ideal gas in void volume, ideal gas in salt/Reactor, BaCl2//NH3, no walls, state-space form, [Tr, Ng, X] as state variables, no algebraic loops, ideal gas in void volume/Reactor, no walls, state space form ==
  q reactor → wall (W) : Inport
  enthalpy_in (J/mol) (only if dn_gas > 0) : Inport  Port=2
  In3 : Inport  Port=3
  Demux : Demux
  Initial condition vector : Constant  Value=[Tr_init; (N_gas_free_volume_init+nu*N_salt*X_init); X_init]
  Integrator1 : Integrator  InitialConditionSource=external
  Mux : Mux  Inputs=3
  Reactor output function : Subsystem
  Reactor state-space functions : Subsystem
  X (0..1) : Outport
  Reactor phase : Outport  Port=2
  P_reactor (bar) : Outport  Port=3
  T_reactor (K) : Outport  Port=4
  h_reactor_free_volume (J/mol) : Outport  Port=5
  wires:
  Reactor output function/1(Out1) -> Demux/1  "Y"
  Reactor output function/2(Out2) -> h_reactor_free_volume (J/mol)/1  "Reactor phase"
  Demux/4 -> T_reactor (K)/1  "h gas free volume (J/mol)"
  Initial condition vector/1 -> Integrator1/2
  Demux/1 -> X (0..1)/1  "T (K)"
  Integrator1/1 -> Reactor output function/1(In1), Reactor state-space functions/1(In1)  "X"
  Demux/2 -> Reactor phase/1  "P (bar)"
  Demux/3 -> P_reactor (bar)/1  "X (0..1)"
  q reactor → wall (W)/1 -> Mux/3  "Q out→in (W)"
  In3/1 -> Mux/2  "h gas in (J/mol)"
  enthalpy_in (J/mol) (only if dn_gas > 0)/1 -> Mux/1  "dn/dt gas (mol/sec) > 0: gas in   < 0: gas out"
  Mux/1 -> Reactor state-space functions/2(In2)
  Reactor state-space functions/1(Out2) -> Integrator1/1

== system thermochemical/Reactors/Reactor, BaCl2//NH3, state-space form, [Tr, Ng, X] as state variables, no algebraic loops, real gas in void volume, ideal gas in salt/Reactor, BaCl2//NH3, no walls, state-space form, [Tr, Ng, X] as state variables, no algebraic loops, real gas in void volume, ideal gas in salt/Reactor, no walls, state space form ==
  q reactor → wall (W) : Inport
  enthalpy_in (J/mol) (only if dn_gas > 0) : Inport  Port=2
  In3 : Inport  Port=3
  Demux : Demux
  Initial condition vector : Constant  Value=[Tr_init; (N_gas_free_volume_init+nu*N_salt*X_init); X_init]
  Integrator1 : Integrator  InitialConditionSource=external
  Mux : Mux  Inputs=3
  Reactor output function : Subsystem
  Reactor state-space functions : Subsystem
  X (0..1) : Outport
  Reactor phase : Outport  Port=2
  P_reactor (bar) : Outport  Port=3
  T_reactor (K) : Outport  Port=4
  h_reactor_free_volume (J/mol) : Outport  Port=5
  wires:
  Reactor state-space functions/1(Out2) -> Integrator1/1
  Mux/1 -> Reactor state-space functions/2(In2)
  enthalpy_in (J/mol) (only if dn_gas > 0)/1 -> Mux/1  "dn/dt gas (mol/sec) > 0: gas in   < 0: gas out"
  In3/1 -> Mux/2  "h gas in (J/mol)"
  q reactor → wall (W)/1 -> Mux/3  "Q out→in (W)"
  Demux/3 -> P_reactor (bar)/1  "X (0..1)"
  Demux/2 -> Reactor phase/1  "P (bar)"
  Integrator1/1 -> Reactor output function/1(In1), Reactor state-space functions/1(In1)  "X"
  Demux/1 -> X (0..1)/1  "T (K)"
  Initial condition vector/1 -> Integrator1/2
  Demux/4 -> T_reactor (K)/1  "h gas free volume (J/mol)"
  Reactor output function/2(Out2) -> h_reactor_free_volume (J/mol)/1  "Reactor phase"
  Reactor output function/1(Out1) -> Demux/1  "Y"

== system thermochemical/Reactors/Reactor, BaCl2//NH3, state-space form, [Tr, Ng, X] as state variables, no algebraic loops, real gas in void volume, real gas in salt/Reactor, BaCl2//NH3, no walls, state-space form, [Tr, Ng, X] as state variables, no algebraic loops, real gas in void volume, real gas in salt/Reactor, no walls, state space form ==
  q reactor → wall (W) : Inport
  enthalpy_in (J/mol) (only if dn_gas > 0) : Inport  Port=2
  In3 : Inport  Port=3
  Demux : Demux
  Initial condition vector : Constant  Value=[Tr_init; (N_gas_free_volume_init+nu*N_salt*X_init); X_init]
  Integrator1 : Integrator  InitialConditionSource=external
  Mux : Mux  Inputs=3
  Reactor output function : Subsystem
  Reactor state-space functions : Subsystem
  X (0..1) : Outport
  Reactor phase : Outport  Port=2
  P_reactor (bar) : Outport  Port=3
  T_reactor (K) : Outport  Port=4
  h_reactor_free_volume (J/mol) : Outport  Port=5
  wires:
  Reactor output function/1(Out1) -> Demux/1  "Y"
  Reactor output function/2(Out2) -> h_reactor_free_volume (J/mol)/1  "Reactor phase"
  Demux/4 -> T_reactor (K)/1  "h gas free volume (J/mol)"
  Initial condition vector/1 -> Integrator1/2
  Demux/1 -> X (0..1)/1  "T (K)"
  Integrator1/1 -> Reactor state-space functions/1(In1), Reactor output function/1(In1)  "X"
  Demux/2 -> Reactor phase/1  "P (bar)"
  Demux/3 -> P_reactor (bar)/1  "X (0..1)"
  q reactor → wall (W)/1 -> Mux/3  "Q out→in (W)"
  In3/1 -> Mux/2  "h gas in (J/mol)"
  enthalpy_in (J/mol) (only if dn_gas > 0)/1 -> Mux/1  "dn/dt gas (mol/sec) > 0: gas in   < 0: gas out"
  Mux/1 -> Reactor state-space functions/2(In2)
  Reactor state-space functions/1(Out2) -> Integrator1/1

== system thermochemical/Reactors/Reactor, BaCl2//NH3, state-space form, [Ur, Ng, X] as state variables, no algebraic loops, ideal gas in void volume, ideal gas in salt/Reactor, BaCl2//NH3, no walls, state-space form, [Ur, Ng, X] as state variables, no algebraic loops, ideal gas in void volume, ideal gas in salt/Reactor, no walls, state space form ==
  q reactor → wall (W) : Inport
  enthalpy_in (J/mol) (only if dn_gas > 0) : Inport  Port=2
  In3 : Inport  Port=3
  Demux : Demux
  Initial conditions : Subsystem
  Integrator1 : Integrator  InitialConditionSource=external
  Mux : Mux  Inputs=3
  Reactor output function : Subsystem
  Reactor state-space functions : Subsystem
  X (0..1) : Outport
  Reactor phase : Outport  Port=2
  P_reactor (bar) : Outport  Port=3
  T_reactor (K) : Outport  Port=4
  h_reactor_free_volume (J/mol) : Outport  Port=5
  wires:
  Reactor output function/1(Out1) -> Demux/1  "Y"
  Reactor output function/2(Out2) -> h_reactor_free_volume (J/mol)/1  "Reactor phase"
  Demux/4 -> T_reactor (K)/1  "h gas free volume (J/mol)"
  Demux/1 -> X (0..1)/1  "T (K)"
  Integrator1/1 -> Reactor state-space functions/1(In1), Reactor output function/1(In1)  "X"
  Demux/2 -> Reactor phase/1  "P (bar)"
  Demux/3 -> P_reactor (bar)/1  "X (0..1)"
  q reactor → wall (W)/1 -> Mux/3  "Q out→in (W)"
  In3/1 -> Mux/2  "h gas in (J/mol)"
  enthalpy_in (J/mol) (only if dn_gas > 0)/1 -> Mux/1  "dn/dt gas (mol/sec) > 0: gas in   < 0: gas out"
  Mux/1 -> Reactor state-space functions/2(In2)
  Reactor state-space functions/1(Out2) -> Integrator1/1
  Initial conditions/1(Out2) -> Integrator1/2

== system thermochemical/Reactors/Reactor, BaCl2//NH3, with algebraic loops, ideal gas in void volume, ideal gas in salt/Reactor, BaCl2//NH3, no walls, with algebraic loops, ideal gas in void volume, ideal gas in salt/Reactor (no walls) ==
  q reactor → wall (W) : Inport
  enthalpy_in (J/mol) (only if dn_gas > 0) : Inport  Port=2
  dn_gas (mol/sec) (if > 0: gas in if < 0: gas out) : Inport  Port=3
  Enthalpy of ideal gas : thermochemical/Thermodynamic fluid properties/Enthalpy of ideal gas  T_ref=T_ref  cP_gas=cP_gas  h_gas_at_T_ref="u_gas_at_T_ref  + R * T_ref"
      settings: SourceProductName=@ Thermochemical
  Integrator8 : Integrator  InitialCondition=N_gas_free_volume_init + X_init*nu*N_salt
  Reactor's internal energy differential equation : Subsystem
  Reactor's temperature and pressure : Subsystem
  T_reactor (K) : Outport
  X (0..1) : Outport  Port=2
  Reactor phase : Outport  Port=3
  h_reactor_free_volume (J/mol) : Outport  Port=4
  P_reactor (bar) : Outport  Port=5
  wires:
  Reactor's temperature and pressure/2(Out1) -> P_reactor (bar)/1  "P_reactor (bar)"
  Reactor's internal energy differential equation/1(Out1) -> Reactor's temperature and pressure/2(In1)
  q reactor → wall (W)/1 -> Reactor's internal energy differential equation/1(In1)  "q out → in (W)"
  Reactor's temperature and pressure/4(Out4) -> X (0..1)/1  "X (0..1)"
  dn_gas (mol/sec) (if > 0: gas in if < 0: gas out)/1 -> Integrator8/1, Reactor's internal energy differential equation/4(In3)  "dn/dt gas (mol/sec) > 0: gas in   < 0: gas out"
  Reactor's temperature and pressure/3(Out2) -> Reactor phase/1  "Reactor phase"
  Reactor's temperature and pressure/1(Out3) -> Enthalpy of ideal gas/1, T_reactor (K)/1  "T_reactor (K)"
  enthalpy_in (J/mol) (only if dn_gas > 0)/1 -> Reactor's internal energy differential equation/2(In2)  "enthalpy in (J/mol) (only if dn/dt gas > 0)"
  Enthalpy of ideal gas/1 -> Reactor's internal energy differential equation/3(In5), h_reactor_free_volume (J/mol)/1  "h gas void space (J/mol)"
  Integrator8/1 -> Reactor's temperature and pressure/1(In2)  "N_gas_reactor"

== system thermochemical/Reactors/Reactor, BaCl2//NH3, with algebraic loops, real gas in void volume, ideal gas in salt/Reactor, BaCl2//NH3, no walls, with algebraic loops, real gas in void volume, ideal gas in salt/Reactor (no walls) ==
  q reactor → wall (W) : Inport
  enthalpy_in (J/mol) (only if dn_gas > 0) : Inport  Port=2
  dn_gas (mol/sec) (if > 0: gas in if < 0: gas out) : Inport  Port=3
  Integrator8 : Integrator  InitialCondition=N_gas_free_volume_init + X_init*nu*N_salt
  Reactor's internal energy differential equation : Subsystem
  Reactor's temperature and pressure : Subsystem
  Thermodynamic property (non-saturated) : thermochemical/Thermodynamic fluid properties/Thermodynamic  property (non-saturated)  sel=h(T,P)  fluid=fluid  reciprocVar=-1  lookup2D_BreakPoint1=fluid.no_sat.T_P_indep.var_indep.T  lookup2D_BreakPoint2=fluid.no_sat.T_P_indep.var_indep.P  lookup2D_Data=fluid.no_sat.T_P_indep.var_dep.h_molar
      settings: SourceProductName=@ Thermochemical
  T_reactor (K) : Outport
  X (0..1) : Outport  Port=2
  Reactor phase : Outport  Port=3
  h_reactor_free_volume (J/mol) : Outport  Port=4
  P_reactor (bar) : Outport  Port=5
  wires:
  Integrator8/1 -> Reactor's temperature and pressure/1(In2)  "N_gas_reactor"
  Thermodynamic property (non-saturated)/1 -> Reactor's internal energy differential equation/3(In5), h_reactor_free_volume (J/mol)/1  "h gas void space (J/mol)"
  enthalpy_in (J/mol) (only if dn_gas > 0)/1 -> Reactor's internal energy differential equation/2(In2)  "enthalpy in (J/mol) (only if dn/dt gas > 0)"
  Reactor's temperature and pressure/1(Out3) -> Thermodynamic property (non-saturated)/1, T_reactor (K)/1  "T_reactor (K)"
  Reactor's temperature and pressure/3(Out2) -> Reactor phase/1  "Reactor phase"
  dn_gas (mol/sec) (if > 0: gas in if < 0: gas out)/1 -> Reactor's internal energy differential equation/4(In3), Integrator8/1  "dn/dt gas (mol/sec) > 0: gas in   < 0: gas out"
  Reactor's temperature and pressure/4(Out4) -> X (0..1)/1  "X (0..1)"
  q reactor → wall (W)/1 -> Reactor's internal energy differential equation/1(In1)  "q out → in (W)"
  Reactor's internal energy differential equation/1(Out1) -> Reactor's temperature and pressure/2(In1)
  Reactor's temperature and pressure/2(Out1) -> Thermodynamic property (non-saturated)/2, P_reactor (bar)/1  "P_reactor (bar)"

== system thermochemical/Reactors/Reactor, BaCl2//NH3, with algebraic loops, real gas in void volume, real gas in salt/Reactor, BaCl2//NH3, no walls, with algebraic loops, real gas in void volume, real gas in salt/Reactor (no walls) ==
  q reactor → wall (W) : Inport
  enthalpy_in (J/mol) (only if dn_gas > 0) : Inport  Port=2
  dn_gas (mol/sec) (if > 0: gas in if < 0: gas out) : Inport  Port=3
  Integrator8 : Integrator  InitialCondition=N_gas_free_volume_init + X_init*nu*N_salt
  Reactor's internal energy differential equation : Subsystem
  Reactor's temperature and pressure : Subsystem
  Thermodynamic property (non-saturated) : thermochemical/Thermodynamic fluid properties/Thermodynamic  property (non-saturated)  sel=h(T,P)  fluid=fluid  reciprocVar=-1  lookup2D_BreakPoint1=fluid.no_sat.T_P_indep.var_indep.T  lookup2D_BreakPoint2=fluid.no_sat.T_P_indep.var_indep.P  lookup2D_Data=fluid.no_sat.T_P_indep.var_dep.h_molar
      settings: SourceProductName=@ Thermochemical
  T_reactor (K) : Outport
  X (0..1) : Outport  Port=2
  Reactor phase : Outport  Port=3
  h_reactor_free_volume (J/mol) : Outport  Port=4
  P_reactor (bar) : Outport  Port=5
  wires:
  Reactor's temperature and pressure/2(Out1) -> P_reactor (bar)/1, Thermodynamic property (non-saturated)/2  "P_reactor (bar)"
  Reactor's internal energy differential equation/1(Out1) -> Reactor's temperature and pressure/2(In1)
  q reactor → wall (W)/1 -> Reactor's internal energy differential equation/1(In1)  "q out → in (W)"
  Reactor's temperature and pressure/4(Out4) -> X (0..1)/1  "X (0..1)"
  dn_gas (mol/sec) (if > 0: gas in if < 0: gas out)/1 -> Integrator8/1, Reactor's internal energy differential equation/4(In3)  "dn/dt gas (mol/sec) > 0: gas in   < 0: gas out"
  Reactor's temperature and pressure/3(Out2) -> Reactor phase/1  "Reactor phase"
  Reactor's temperature and pressure/1(Out3) -> T_reactor (K)/1, Thermodynamic property (non-saturated)/1  "T_reactor (K)"
  enthalpy_in (J/mol) (only if dn_gas > 0)/1 -> Reactor's internal energy differential equation/2(In2)  "enthalpy in (J/mol) (only if dn/dt gas > 0)"
  Thermodynamic property (non-saturated)/1 -> h_reactor_free_volume (J/mol)/1, Reactor's internal energy differential equation/3(In5)  "h gas void space (J/mol)"
  Integrator8/1 -> Reactor's temperature and pressure/1(In2)  "N_gas_reactor"

== system thermochemical/Valves/Valve, gas, IEC 60534-2-1:2012 (exact)/Flow computation for compressible fluids, IEC 60534-2-1:2012/Subsystem ==
  P downstream (bar) : Inport
  P upstream (bar) : Inport  Port=2
  P upstream (bar)1 : Inport  Port=3
  Display{1..5} (5 alike) : Display
  Divide : Product  Inputs=*/
  Divide2 : Product  Inputs=*/
  Gain2 : Gain  Gain=xT
  "Heat capacity ratio of air @ (60°F, 1atm)" : Constant  Value=1.40
  Sign : Signum
  Sum3 : Sum  Inputs=-+
  Sum4 : Sum  Inputs=-+
  Switch1 : Switch  Criteria=u2 > Threshold
  non-chocked : Outport
  non-chocked2 : Outport  Port=2
  non-chocked1 : Outport  Port=3
  wires:
  Switch1/1 -> Display5/1, non-chocked2/1  "x sizing"
  P upstream (bar)/1 -> Divide2/2, Sum3/2  "P upstream (bar)"
  P downstream (bar)/1 -> Sum3/1  "P downstream (bar)"
  Sign/1 -> Switch1/2, Display4/1, non-chocked/1  "non-chocked"
  Gain2/1 -> Switch1/3, Display2/1, non-chocked1/1, Sum4/2  "x chocked"
  Sum4/1 -> Sign/1
  Sum3/1 -> Divide2/1  "dP"
  Divide2/1 -> Display3/1, Sum4/1, Switch1/1  "x"
  P upstream (bar)1/1 -> Divide/1  "gamma upstream"
  "Heat capacity ratio of air @ (60°F, 1atm)"/1 -> Divide/2  "gamma air"
  Divide/1 -> Display1/1, Gain2/1  "Fgamma"

== system thermochemical/Valves/Valve, gas, IEC 60534-2-1:2012 (exact)/Flow computation for compressible fluids, IEC 60534-2-1:2012/Subsystem1 ==
  In1 : Inport
  In2 : Inport  Port=2
  Constant : Constant
  Display4 : Display
  Divide : Product  Inputs=*/
  Gain : Gain  Gain=3
  Sum3 : Sum  Inputs=+-|
  Y : Outport
  wires:
  Divide/1 -> Sum3/2
  In2/1 -> Gain/1  "x chocked"
  Sum3/1 -> Display4/1, Y/1  "Y"
  Gain/1 -> Divide/2
  In1/1 -> Divide/1  "x sizing"
  Constant/1 -> Sum3/1
